simulink model "am_sys3"  (Simulink 3.00)
settings: Solver=ode45  StartTime=0.0  StopTime=1000  MaxStep=0.001  RelTol=1e-3  AbsTol=1e-3
undefined symbols (not defined in the file): at, bt, ct, dt
settings Model: SaveTime=off  SaveOutput=off

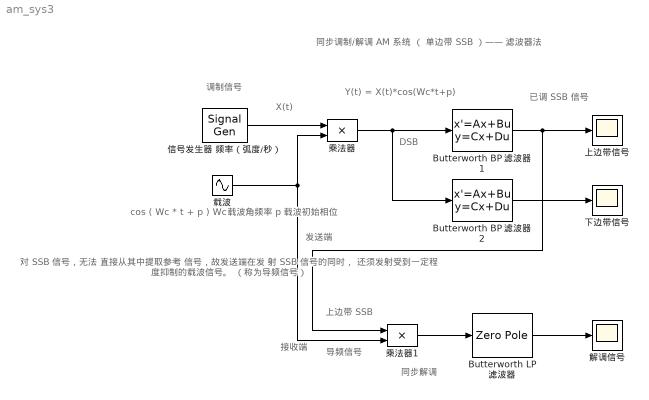
== system am_sys3 ==
  note: 同步解调
  note: 同步调制/解调 AM 系统 （ 单边带 SSB ）—— 滤波器法
  note: 上边带 SSB
  note: 导频信号
  note: DSB
  note: cos ( Wc * t + p )
      | Wc 载波角频率
      | p 载波初始相位
  note: 调制信号
  note: X(t)
  note: Y(t) = X(t)*cos(Wc*t+p)
  note: 已调 SSB 信号
  note: 对 SSB 信号，无法
      | 直接从其中提取参考
      | 信号，故发送端在发
      | 射 SSB 信号的同时，
      | 还须发射受到一定程
      | 度抑制的载波信号。
      | （称为导频信号）
  note: 发送端
  note: 接收端
  Butterworth BP 滤波器 1 : StateSpace  A=at  B=bt  C=ct  D=dt  X0=0  mask(buttap,lp2bp){@1=110, @2=5, @3=4}
      mask prompts: @1 "Center frequency (rad/sec)"; @2 "Bandwidth (rad/sec):"; @3 "Order"
      mask help:
      | Analog Butterworth band pass filter.
      |
      | (Requires Signal Processing Toolbox)
      mask init:
      | [at,bt,ct,dt,w,mag]=filtm('buttap','lp2bp',@1,@2,50,@3);
      mask Help: Butterworth band pass filter using MATLAB's butter and lp2bp command.
      mask Display: plot(w,mag)
  Butterworth BP 滤波器 2 : StateSpace  A=at  B=bt  C=ct  D=dt  X0=0  mask(buttap,lp2bp){@1=90, @2=5, @3=4}
      mask prompts: @1 "Center frequency (rad/sec)"; @2 "Bandwidth (rad/sec):"; @3 "Order"
      mask help:
      | Analog Butterworth band pass filter.
      |
      | (Requires Signal Processing Toolbox)
      mask init:
      | [at,bt,ct,dt,w,mag]=filtm('buttap','lp2bp',@1,@2,50,@3);
      mask Help: Butterworth band pass filter using MATLAB's butter and lp2bp command.
      mask Display: plot(w,mag)
  Butterworth LP 滤波器 : ZeroPole  Zeros=z  Poles=p  Gain=k  mask(buttap){@1=15, @2=4}
      mask prompts: @1 "Cutoff frequency (rad/sec)"; @2 "Order"
      mask help:
      | Analog Butterworth low pass filter.
      |
      | (Requires Signal Processing Toolbox)
      mask init:
      | [z,p,k]=buttap(@2); z=@1*z; p=@1*p; k=real(prod(-p)); [num,den]=zp2tf(z,p,k); w=logspace(log10(@1/10),log10(10*@1),20); h=freqs(num,den,w);
      mask Help: Butterworth low pass filter using MATLAB's butter command.
      mask Display: plot(20*log10(w),20*log10(abs(h)))
  乘法器 : Product  Inputs=2  SaturateOnIntegerOverflow=on
      mask Type: 乘法器
      mask Description: 乘法器
      mask Display: plot([0 1],[1 0],[0 1],[0 1]);
  乘法器1 : Product  Inputs=2  SaturateOnIntegerOverflow=on
      mask Type: 乘法器
      mask Description: 乘法器
      mask Display: plot([0 1],[1 0],[0 1],[0 1]);
  解调信号 : Scope
      settings: TimeRange=1.000000  YMin=-1  YMax=1  SaveToWorkspace=off  SaveName=ScopeData  DataFormat=Matrix
  上边带信号 : Scope
      settings: TimeRange=1.000000  YMin=-2  YMax=2  SaveToWorkspace=off  SaveName=ScopeData  DataFormat=Matrix
  下边带信号 : Scope
      settings: TimeRange=1.000000  YMin=-2  YMax=2  SaveToWorkspace=off  SaveName=ScopeData  DataFormat=Matrix
  信号发生器 频率（弧度/秒） : SignalGenerator  WaveForm=sine  Amplitude=1.000000  Frequency=10.000000  Units=rad/sec
  载波 : Sin  Amplitude=1  Frequency=100  Phase=0  SampleTime=0.001
  wires:
  Butterworth LP 滤波器/1 -> 解调信号/1
  乘法器1/1 -> Butterworth LP 滤波器/1
  Butterworth BP 滤波器 1/1 -> 上边带信号/1, 乘法器1/1
  载波/1 -> 乘法器/2, 乘法器1/2
  Butterworth BP 滤波器 2/1 -> 下边带信号/1
  乘法器/1 -> Butterworth BP 滤波器 1/1, Butterworth BP 滤波器 2/1
  信号发生器 频率（弧度/秒）/1 -> 乘法器/1
